simulink subsystem "disable_integrator_on_start_up"  (R2020b)
settings: Solver=VariableStepAuto  StartTime=0.0  StopTime=10.0  RelTol=1e-3
libraries: simulink x1
settings Model: Creator=unix  LastModifiedBy=unix

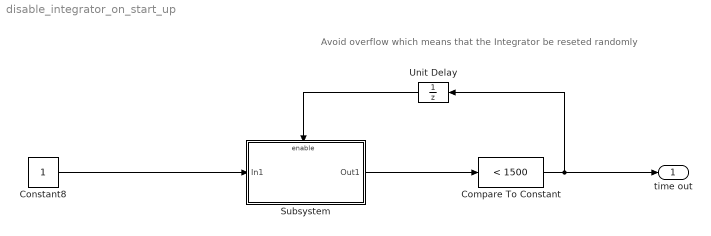
== system disable_integrator_on_start_up ==
  note: Avoid overflow which means that the Integrator be reseted randomly
  Compare To Constant : simulink/Logic and Bit Operations/Compare To Constant  relop=<  const=1500  OutDataTypeStr=boolean
  Constant8 : Constant  OutDataTypeStr=uint8
  Subsystem : Subsystem
  Unit Delay : UnitDelay  SampleTime=-1  HasFrameUpgradeWarning=on
  time out : Outport
  wires:
  Compare To Constant/1 -> time out/1, Unit Delay/1
  Subsystem/1(Out1) -> Compare To Constant/1
  Constant8/1 -> Subsystem/1(In1)
  Unit Delay/1 -> Subsystem/Enable

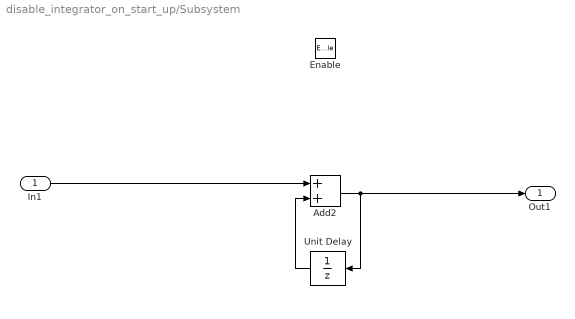
== system disable_integrator_on_start_up/Subsystem ==
  In1 : Inport
  Enable : EnablePort  PropagateVarSize=During execution
  Add2 : Sum  OutDataTypeStr=uint16
  Unit Delay : UnitDelay  SampleTime=-1  HasFrameUpgradeWarning=on
  Out1 : Outport
  wires:
  Add2/1 -> Unit Delay/1, Out1/1
  In1/1 -> Add2/1
  Unit Delay/1 -> Add2/2
